simulink model "fan_model_c"  (R2024b)
settings: Solver=VariableStepAuto  StartTime=0.0  StopTime=100  FixedStep=1e-4  RelTol=1e-6
values from neighbouring files (symbols this model uses):
  a = 0.0    [data.sldd]
  J_f = 0.0    [data.sldd]
  J_m = 0.0    [data.sldd]
  RateSpeed = 0.0    [data.sldd]
  Speed_max = 0.0    [data.sldd]
  T0 = 0.0    [data.sldd]
  Torque_max = 0.0    [data.sldd]
settings Model: DataDictionary=data.sldd  Creator=SESA504213  LastModifiedBy=SESA504213

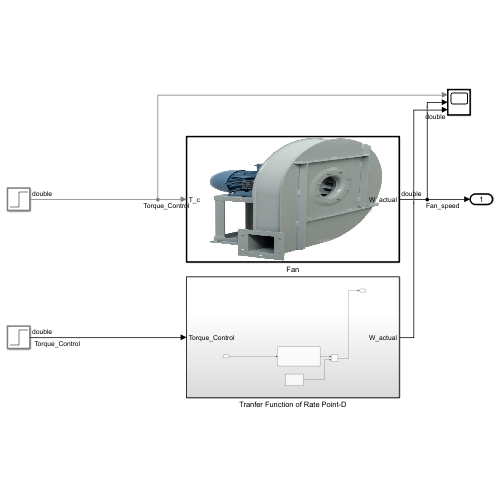
[thumbnail: Simulink's stored preview of the top-level diagram]
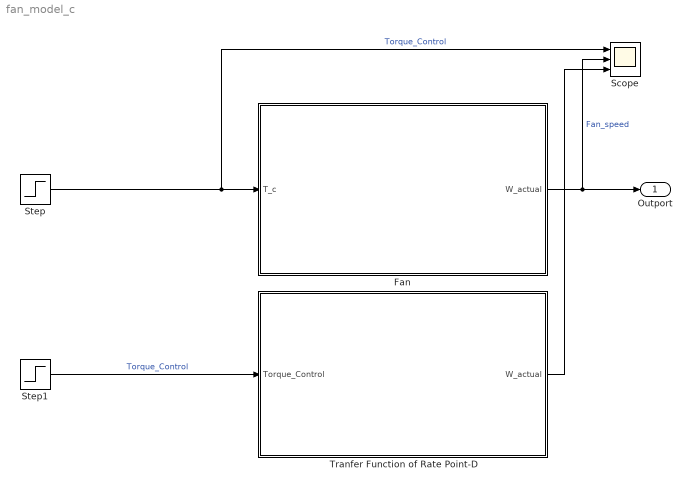
== system fan_model_c ==
  Fan : Subsystem
      mask Display: image('FanwithMotor.jpg');
  Scope : Scope  NumInputPorts=3
  Step : Step  Time=50  Before=13.126  After=16.12  SampleTime=0
  Step1 : Step  Time=50  After=3  SampleTime=0
  Tranfer Function of Rate Point-D : Subsystem
  Outport : Outport
  wires:
  Fan/1(W_actual) -> Outport/1, Scope/2  "Fan_speed"
  Step/1 -> Scope/1, Fan/1(T_c)  "Torque_Control"
  Step1/1 -> Tranfer Function of Rate Point-D/1(Torque_Control)  "Torque_Control"
  Tranfer Function of Rate Point-D/1(W_actual) -> Scope/3

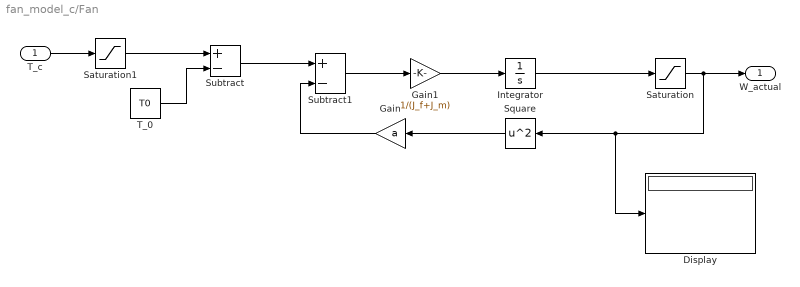
== system fan_model_c/Fan ==
  T_c : Inport
  Display : Display
  Gain : Gain  Gain=a
  Gain1 : Gain  Gain=1/(J_f+J_m)
  Integrator : Integrator
  Saturation : Saturate  UpperLimit=Speed_max  LowerLimit=-Speed_max
  Saturation1 : Saturate  UpperLimit=Torque_max  LowerLimit=-Torque_max
  Square : Math  Operator=square
  Subtract : Sum  Inputs=+-
  Subtract1 : Sum  Inputs=+-
  T_0 : Constant  Value=T0
  W_actual : Outport
  wires:
  Gain1/1 -> Integrator/1
  Square/1 -> Gain/1
  T_c/1 -> Saturation1/1
  T_0/1 -> Subtract/2
  Subtract1/1 -> Gain1/1
  Integrator/1 -> Saturation/1
  Subtract/1 -> Subtract1/1
  Gain/1 -> Subtract1/2
  Saturation/1 -> Display/1, Square/1, W_actual/1
  Saturation1/1 -> Subtract/1

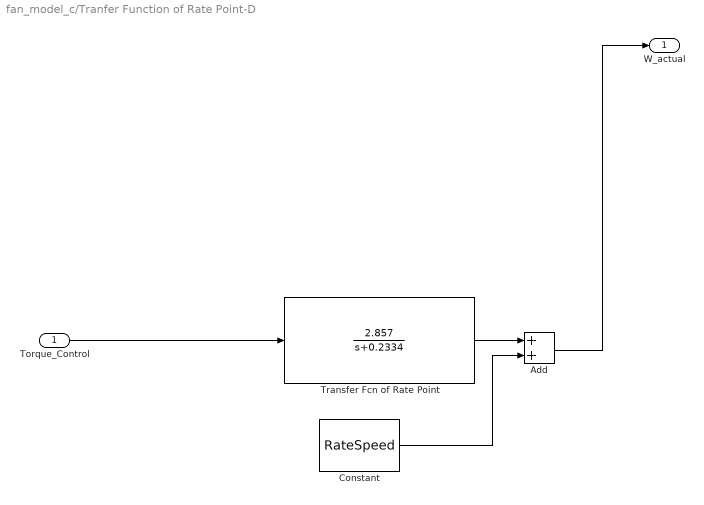
== system fan_model_c/Tranfer Function of Rate Point-D ==
  Torque_Control : Inport
  Add : Sum
  Constant : Constant  Value=RateSpeed
  "Transfer Fcn of Rate Point " : TransferFcn  Numerator=[2.857]  Denominator=[1 0.2334]
  W_actual : Outport
  wires:
  "Transfer Fcn of Rate Point "/1 -> Add/1
  Constant/1 -> Add/2
  Torque_Control/1 -> "Transfer Fcn of Rate Point "/1
  Add/1 -> W_actual/1
